simulink model "lee_controller"  (R2021b)
settings: Solver=FixedStepAuto  StartTime=0.0  StopTime=inf  FixedStep=dt  RelTol=1e-3  EnableMultiTasking=on
values from neighbouring files (symbols this model uses):
  dt = 1/250    (= 0.004)    [parameters.m]
  ei = [0,0,0]'    [parameters.m]
  eir = [0,0,0]'    [parameters.m]
  g = 9.81    [parameters.m]
  pitch_offset = 0.028    [parameters.m]
  roll_offset = 0.028    [parameters.m]
  thrust_offset = 0.075    [parameters.m]
  yaw_offset = 0.028    [parameters.m]
undefined symbols (not defined in the file or in its folder): AUX, ddz, dev, DiscIntNeverNeededParam, dz, ep, ev, ew, eyaw, f_ext, fz, Main, pwm_output0, pwm_output1, tau, timestamp, z
libraries: px4lib x47, px4uORBlib x14, px4Sensorslib x1
(part 1 of 2)
settings Model: SimulationMode=external  ExtModeTrigDuration=10  Creator=salvatore  LastModifiedBy=simone
settings SolverCC: PositivePriorityOrder=on
settings DataIOCC: MaxDataPoints=7018
settings OptimizationCC: EnhancedBackFolding=on  PassReuseOutputArgsAs=Individual arguments  ZeroExternalMemoryAtStartup=off  ZeroInternalMemoryAtStartup=off  MaxStackSize=64  OptimizeBlockOrder=speed  DifferentSizesBufferReuse=on  OptimizationCustomize=off  EfficientTunableParamExpr=on
settings DebuggingCC: ParameterTunabilityLossMsg=error
settings HardwareCC: ProdBitPerPointer=32  ProdBitPerSizeT=32  ProdBitPerPtrDiffT=32  ProdLargestAtomicInteger=Long  ProdLargestAtomicFloat=Double  ProdWordSize=32  ProdLongLongMode=on  ProdHWDeviceType=ARM Compatible->ARM Cortex
settings SFSimCC: MATLABDynamicMemAlloc=off  SimTargetLang=C++
settings RTWCC: Description=Embedded Coder  SystemTargetFile=ert.tlc  HardwareBoard=PX4 Pixhawk 4  TLCOptions="-aInlineSetEventsForThisBaseRateFcn=TLC_FALSE -aSuppressMultiTaskScheduler=TLC_FALSE  -aRateBasedStepFcn=0"  TemplateMakefile=ert_default_tmf  Toolchain=GNU Tools for PX4 Autopilots  TargetLang=C++
settings CodeAppCC: ForceParamTrailComments=on  IgnoreCustomStorageClasses=off  OperatorAnnotations=on  SimulinkDataObjDesc=on  SFDataObjDesc=on  InsertBlockDesc=on
settings ERTTargetCC: ExtMode=on  ExtModeTransport=3  ExtModeStaticAlloc=on  ExtModeStaticAllocSize=1024  ExtModeMexFile=ext_xcp  ExtModeMexArgs=1 /dev/ttyUSB0 115200  ExtModeIntrfLevel=Level2 - Open

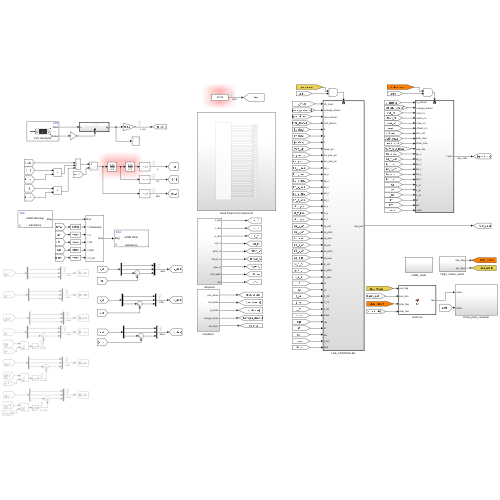
[thumbnail: Simulink's stored preview of the top-level diagram]
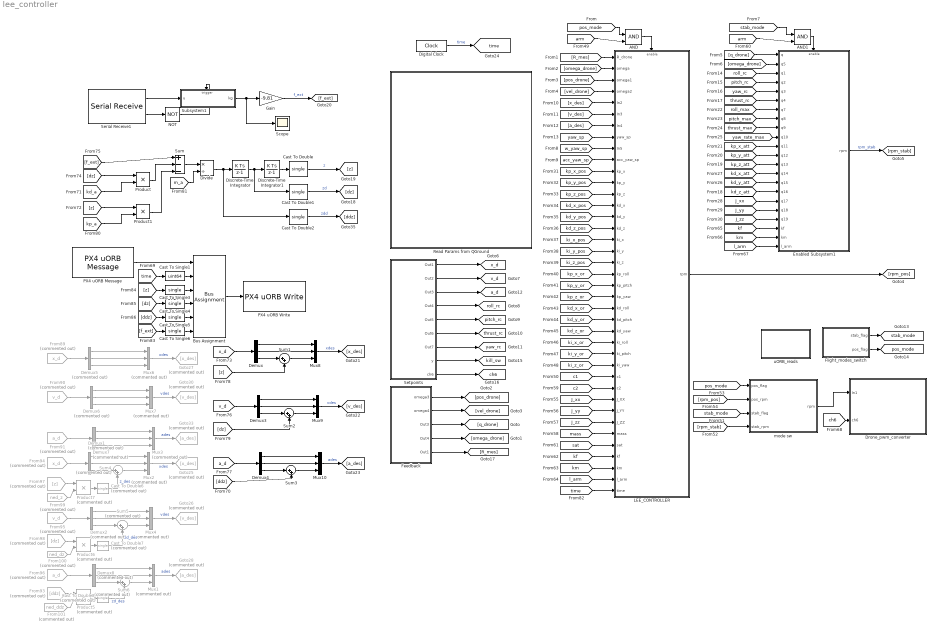
== system lee_controller ==
  AND : Logic  IconShape=distinctive  AllPortsSameDT=off  OutDataTypeStr=boolean
  AND1 : Logic  IconShape=distinctive  AllPortsSameDT=off  OutDataTypeStr=boolean
  Bus Assignment : BusAssignment  AssignedSignals=timestamp,z,dz,ddz,f_ext
  Cast To Double : DataTypeConversion  OutDataTypeStr=single
  Cast To Double1 : DataTypeConversion  OutDataTypeStr=single
  Cast To Double2 : DataTypeConversion  OutDataTypeStr=single
  Cast To Double6 : DataTypeConversion  Commented=on  OutDataTypeStr=single
  Cast To Double7 : DataTypeConversion  Commented=on  OutDataTypeStr=single
  Cast To Double8 : DataTypeConversion  Commented=on  OutDataTypeStr=single
  Cast To Single1 : DataTypeConversion  OutDataTypeStr=uint64
  Cast To Single{3..6} (4 alike) : DataTypeConversion  OutDataTypeStr=single
  Demux : Demux  Outputs=3
  Demux{1..2,5..8} (6 alike) : Demux  Commented=on  Outputs=3
  Demux3 : Demux  Outputs=3
  Demux4 : Demux  Outputs=3
  Digital Clock : DigitalClock  SampleTime=dt
  Discrete-Time Integrator : DiscreteIntegrator  SampleTime=dt  OutDataTypeStr=double  ICPrevOutput=DiscIntNeverNeededParam  ICPrevScaledInput=DiscIntNeverNeededParam
  Discrete-Time Integrator1 : DiscreteIntegrator  SampleTime=dt  OutDataTypeStr=double  ICPrevOutput=DiscIntNeverNeededParam  ICPrevScaledInput=DiscIntNeverNeededParam
  Divide : Product  Inputs=*/  OutDataTypeStr=double
  Drone_pwm_converter : Subsystem
  Enabled Subsystem1 : Subsystem  TreatAsAtomicUnit=on
  Feedback : Subsystem
  Flight_modes_switch : Subsystem
  From100 : From  Commented=on  GotoTag=ned_dz  TagVisibility=global
  From101 : From  Commented=on  GotoTag=ned_ddz  TagVisibility=global
  From89 : From  Commented=on  GotoTag=x_d  TagVisibility=global
  From90 : From  Commented=on  GotoTag=v_d  TagVisibility=global
  From91 : From  Commented=on  GotoTag=a_d  TagVisibility=global
  From93 : From  Commented=on  GotoTag=ddz
  From94 : From  Commented=on  GotoTag=x_d  TagVisibility=global
  From95 : From  Commented=on  GotoTag=v_d  TagVisibility=global
  From96 : From  Commented=on  GotoTag=a_d  TagVisibility=global
  From97 : From  Commented=on  GotoTag=z
  From98 : From  Commented=on  GotoTag=dz
  From99 : From  Commented=on  GotoTag=ned_z  TagVisibility=global
  Gain : Gain  Gain=-9.81
  Goto25 : Goto  Commented=on  GotoTag=x_des
  Goto26 : Goto  Commented=on  GotoTag=v_des
  Goto27 : Goto  Commented=on  GotoTag=x_des
  Goto28 : Goto  Commented=on  GotoTag=a_des
  Goto30 : Goto  Commented=on  GotoTag=v_des
  Goto33 : Goto  Commented=on  GotoTag=a_des
  LEE_CONTROLLER : Subsystem  TreatAsAtomicUnit=on
  Mux{1..4,6..7} (6 alike) : Mux  Commented=on  Inputs=3
  Mux10 : Mux  Inputs=3
  Mux8 : Mux  Inputs=3
  Mux9 : Mux  Inputs=3
  NOT : Logic  Operator=NOT  IconShape=distinctive  AllPortsSameDT=off  OutDataTypeStr=boolean
  PX4 uORB Message : px4uORBlib/PX4 uORB Message  uORBTopic=admittance  SampleTime=dt  selectInstance=admittance
      settings: SourceProductBaseCode=PX4AUTOPILOTS
  PX4 uORB Write : px4uORBlib/PX4 uORB Write  uORBTopic=admittance  selectInstance=admittance  MessageQueueLen=1
      settings: SourceProductBaseCode=PX4AUTOPILOTS
  Product : Product
  Product1 : Product
  Product5 : Product  Commented=on
  Product6 : Product  Commented=on
  Product7 : Product  Commented=on
  Read Params from QGround : Subsystem
  Scope : Scope
  Serial Receive1 : px4lib/Serial Receive  SCIModule=/dev/ttyS2  DataType=int8  DataLength=2  OutputStatus=on  SampleTime=dt  BlockingMode=off  PartialData=off  Timeout=5
      settings: SourceProductBaseCode=PX4AUTOPILOTS
  Setpoints : Subsystem
  Subsystem1 : Subsystem
  Sum : Sum  Inputs=|+--
  Sum1 : Sum  Inputs=|++
  Sum2 : Sum  Inputs=|++
  Sum3 : Sum  Inputs=|++
  Sum4 : Sum  Commented=on  Inputs=|++
  Sum5 : Sum  Commented=on  Inputs=|++
  Sum6 : Sum  Commented=on  Inputs=|++
  mode sw : MATLAB Function  TreatAsAtomicUnit=on
  uORB_reads : Subsystem
  tag scope: a_d=global, ch6=global, kill_sw=global, pitch_rc=global, pos_mode=global, roll_rc=global, stab_mode=global, thrust_rc=global, time=global, v_d=global, x_d=global, yaw_rc=global
  wires:
  [omega_drone] -> LEE_CONTROLLER/2(omega)
  [pos_drone] -> LEE_CONTROLLER/3(omega1)
  [vel_drone] -> LEE_CONTROLLER/4(omega2)
  [omega_drone] -> Enabled Subsystem1/2(q5)
  Enabled Subsystem1/1(rpm) -> [rpm_stab]  "rpm_stab"
  [x_des] -> LEE_CONTROLLER/5(In2)
  [v_des] -> LEE_CONTROLLER/6(In3)
  [a_des] -> LEE_CONTROLLER/7(In4)
  Setpoints/2(Out2) -> [v_d]
  Setpoints/1(Out1) -> [x_d]
  Setpoints/3(Out3) -> [a_d]
  Setpoints/4(Out4) -> [roll_rc]
  Setpoints/5(Out5) -> [pitch_rc]
  Setpoints/7(Out7) -> [yaw_rc]
  Setpoints/6(Out6) -> [thrust_rc]
  [roll_rc] -> Enabled Subsystem1/3(q1)
  [pitch_rc] -> Enabled Subsystem1/4(q2)
  [yaw_rc] -> Enabled Subsystem1/5(q3)
  [thrust_rc] -> Enabled Subsystem1/6(q4)
  Flight_modes_switch/1(stab_flag) -> [stab_mode]
  Flight_modes_switch/2(pos_flag) -> [pos_mode]
  [q_drone] -> Enabled Subsystem1/1(q)
  Setpoints/8(y) -> [kill_sw]
  [roll_max] -> Enabled Subsystem1/7(q7)
  [pitch_max] -> Enabled Subsystem1/8(q8)
  [thrust_max] -> Enabled Subsystem1/9(q9)
  [yaw_rate_max] -> Enabled Subsystem1/10(q10)
  [kp_x_att] -> Enabled Subsystem1/11(q11)
  [kp_y_att] -> Enabled Subsystem1/12(q12)
  [kp_z_att] -> Enabled Subsystem1/13(q13)
  [kd_x_att] -> Enabled Subsystem1/14(q14)
  [kd_y_att] -> Enabled Subsystem1/15(q15)
  [kd_z_att] -> Enabled Subsystem1/16(q16)
  [J_zz] -> Enabled Subsystem1/19(q19)
  [J_yy] -> Enabled Subsystem1/18(q18)
  [J_xx] -> Enabled Subsystem1/17(q17)
  [kp_x_pos] -> LEE_CONTROLLER/11(kp_x)
  [kp_y_pos] -> LEE_CONTROLLER/12(kp_y)
  [kp_z_pos] -> LEE_CONTROLLER/13(kp_z)
  [kd_x_pos] -> LEE_CONTROLLER/14(kd_x)
  [kd_y_pos] -> LEE_CONTROLLER/15(kd_y)
  [kd_z_pos] -> LEE_CONTROLLER/16(kd_z)
  [ki_x_pos] -> LEE_CONTROLLER/17(ki_x)
  [ki_y_pos] -> LEE_CONTROLLER/18(ki_y)
  [ki_z_pos] -> LEE_CONTROLLER/19(ki_z)
  [kp_x_or] -> LEE_CONTROLLER/20("kp_roll\t")
  [kp_y_or] -> LEE_CONTROLLER/21(kp_pitch)
  [kp_z_or] -> LEE_CONTROLLER/22(kp_yaw)
  [kd_x_or] -> LEE_CONTROLLER/23(kd_roll)
  [kd_y_or] -> LEE_CONTROLLER/24(kd_pitch)
  [kd_z_or] -> LEE_CONTROLLER/25(kd_yaw)
  [ki_x_or] -> LEE_CONTROLLER/26(ki_roll)
  [ki_y_or] -> LEE_CONTROLLER/27(ki_pitch)
  [ki_z_or] -> LEE_CONTROLLER/28(ki_yaw)
  [c1] -> LEE_CONTROLLER/29(c1)
  [stab_mode] -> mode sw/3(stab_flag)
  [rpm_stab] -> mode sw/4(stab_rpm)
  [rpm_pos] -> mode sw/2(pos_rpm)
  [pos_mode] -> mode sw/1(pos_flag)
  mode sw/1(rpm) -> Drone_pwm_converter/1(In1)
  [J_yy] -> LEE_CONTROLLER/32(J_YY)
  [J_xx] -> LEE_CONTROLLER/31(J_XX)
  [J_zz] -> LEE_CONTROLLER/33(J_ZZ)
  [c2] -> LEE_CONTROLLER/30(c2)
  [mass] -> LEE_CONTROLLER/34("mass ")
  Feedback/1(omega3) -> [pos_drone]
  Feedback/3(Out3) -> [q_drone]
  Feedback/4(Out4) -> [omega_drone]
  Feedback/2(omega4) -> [vel_drone]
  [yaw_sp] -> LEE_CONTROLLER/8(yaw_sp)
  [w_yaw_sp] -> LEE_CONTROLLER/9(In5)
  [acc_yaw_sp] -> LEE_CONTROLLER/10(acc_yaw_sp)
  Feedback/5(Out1) -> [R_mes]
  [R_mes] -> LEE_CONTROLLER/1(R_drone)
  LEE_CONTROLLER/1(rpm) -> [rpm_pos]
  AND/1 -> LEE_CONTROLLER/Enable
  [pos_mode] -> AND/1
  [arm] -> AND/2
  AND1/1 -> Enabled Subsystem1/Enable
  [arm] -> AND1/2
  [stab_mode] -> AND1/1
  [sat] -> LEE_CONTROLLER/35(sat)
  [kf] -> LEE_CONTROLLER/36(kf)
  [km] -> LEE_CONTROLLER/37(km)
  [l_arm] -> LEE_CONTROLLER/38(l_arm)
  [kf] -> Enabled Subsystem1/20(kf)
  [km] -> Enabled Subsystem1/21(km)
  [l_arm] -> Enabled Subsystem1/22(l_arm)
  Setpoints/9(ch6) -> [ch6]
  [ch6] -> Drone_pwm_converter/2(ch6)
  Sum1/1 -> Mux8/3
  Demux3/3 -> Sum2/1
  Demux4/1 -> Mux10/1
  [m_a] -> Divide/2
  [f_ext] -> Sum/1
  Demux/1 -> Mux8/1
  Gain/1 -> [f_ext]  "f_ext"
  Sum3/1 -> Mux10/3
  Divide/1 -> Cast To Double2/1, Discrete-Time Integrator/1
  [dz] -> Product/1
  NOT/1 -> Subsystem1/Trigger
  Serial Receive1/2 -> NOT/1
  Sum2/1 -> Mux9/3
  [x_d] -> Demux/1
  Mux10/1 -> [a_des]  "ades"
  Discrete-Time Integrator/1 -> Discrete-Time Integrator1/1, Cast To Double1/1
  Demux/2 -> Mux8/2
  Cast To Single3/1 -> Bus Assignment/3
  [dz] -> Cast To Single4/1
  Sum/1 -> Divide/1
  Cast To Single4/1 -> Bus Assignment/4
  Demux3/1 -> Mux9/1
  [z] -> Cast To Single3/1
  Cast To Single5/1 -> Bus Assignment/5
  [a_d] -> Demux4/1
  Demux4/3 -> Sum3/1
  Subsystem1/1(kg) -> Scope/1, Gain/1
  Bus Assignment/1 -> PX4 uORB Write/1
  Demux4/2 -> Mux10/2
  [ddz] -> Cast To Single5/1
  Cast To Single6/1 -> Bus Assignment/6
  Demux3/2 -> Mux9/2
  [f_ext] -> Cast To Single6/1
  [kd_a] -> Product/2
  Product/1 -> Sum/2
  Mux8/1 -> [x_des]  "xdes"
  Product1/1 -> Sum/3
  PX4 uORB Message/1 -> Bus Assignment/1
  [z] -> Product1/1
  Mux9/1 -> [v_des]  "vdes"
  [kp_a] -> Product1/2
  Serial Receive1/1 -> Subsystem1/1(u)
  [v_d] -> Demux3/1
  Demux/3 -> Sum1/1
  Demux7/2 -> Mux3/2
  Mux6/1 -> Goto27/1  "xdes"
  From90/1 -> Demux6/1
  Demux5/1 -> Mux6/1
  Demux6/3 -> Mux7/3
  Demux5/2 -> Mux6/2
  From91/1 -> Demux7/1
  Demux7/3 -> Mux3/3
  Mux3/1 -> Goto33/1  "ades"
  Demux6/1 -> Mux7/1
  From89/1 -> Demux5/1
  Demux6/2 -> Mux7/2
  Demux5/3 -> Mux6/3
  Demux7/1 -> Mux3/1
  Mux7/1 -> Goto30/1  "vdes"
  Discrete-Time Integrator1/1 -> Cast To Double/1
  Cast To Double/1 -> [z]  "z"
  Cast To Double1/1 -> [dz]  "zd"
  Cast To Double2/1 -> [ddz]  "zdd"
  Digital Clock/1 -> [time]  "time"
  [time] -> Cast To Single1/1
  Cast To Single1/1 -> Bus Assignment/2
  [time] -> LEE_CONTROLLER/39(time)
  [z] -> Sum1/2
  [dz] -> Sum2/2
  [ddz] -> Sum3/2
  Product5/1 -> Cast To Double8/1
  Product7/1 -> Cast To Double6/1
  Demux8/1 -> Mux1/1
  From93/1 -> Product5/1
  Sum6/1 -> Mux1/3
  From94/1 -> Demux1/1
  Mux4/1 -> Goto26/1  "vdes"
  Cast To Double6/1 -> Sum4/2  "z_des"
  Demux2/2 -> Mux4/2
  Demux8/2 -> Mux1/2
  Product6/1 -> Cast To Double7/1
  Demux1/3 -> Sum4/1
  From97/1 -> Product7/1
  Demux1/2 -> Mux2/2
  From95/1 -> Demux2/1
  From99/1 -> Product7/2
  Sum4/1 -> Mux2/3
  Demux2/1 -> Mux4/1
  From100/1 -> Product6/2
  Sum5/1 -> Mux4/3
  Mux1/1 -> Goto28/1  "ades"
  From98/1 -> Product6/1
  From101/1 -> Product5/2
  Demux2/3 -> Sum5/1
  Cast To Double7/1 -> Sum5/2  "zd_des"
  From96/1 -> Demux8/1
  Cast To Double8/1 -> Sum6/2  "zd_des"
  Demux1/1 -> Mux2/1
  Demux8/3 -> Sum6/1
  Mux2/1 -> Goto25/1  "xdes"

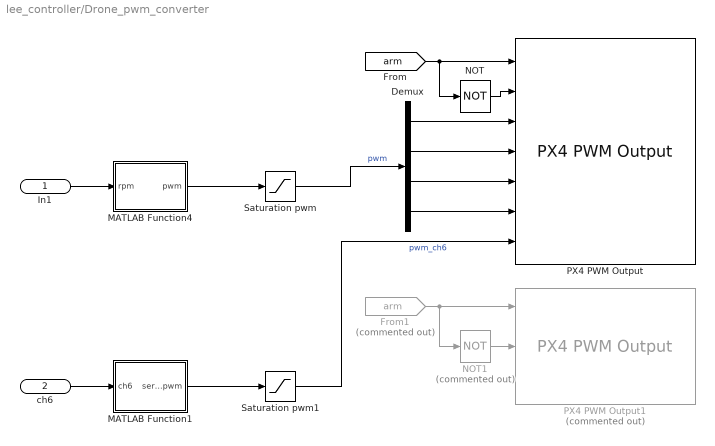
== system lee_controller/Drone_pwm_converter ==
  In1 : Inport
  ch6 : Inport  Port=2
  Demux : Demux
  From1 : From  Commented=on  GotoTag=arm  TagVisibility=global
  MATLAB Function1 : MATLAB Function  TreatAsAtomicUnit=on
  MATLAB Function4 : MATLAB Function  TreatAsAtomicUnit=on
  NOT : Logic  Operator=NOT  IconShape=distinctive  AllPortsSameDT=off  OutDataTypeStr=boolean
  NOT1 : Logic  Commented=on  Operator=NOT  IconShape=distinctive  AllPortsSameDT=off  OutDataTypeStr=boolean
  PX4 PWM Output : px4lib/PX4 PWM Output  pwmDevice=Main (/dev/pwm_output0)  pwmChannel1_=on  pwmChannel2_=on  pwmChannel3_=on  pwmChannel4_=on  pwmChannel5_=off  pwmChannel6_=off  pwmChannel7_=off  pwmChannel8_=on  forceTerminateFailsafe=off  outputErrorStatus=off
      settings: SourceProductBaseCode=PX4AUTOPILOTS
  PX4 PWM Output1 : px4lib/PX4 PWM Output  Commented=on  pwmDevice=AUX (/dev/pwm_output1)  pwmChannel1_=off  pwmChannel2_=off  pwmChannel3_=on  pwmChannel4_=off  pwmChannel5_=off  pwmChannel6_=off  pwmChannel7_=off  pwmChannel8_=off  forceTerminateFailsafe=off  outputErrorStatus=off
      settings: SourceProductBaseCode=PX4AUTOPILOTS
  Saturation pwm : Saturate  UpperLimit=2000  LowerLimit=1000  LinearizeAsGain=off
  Saturation pwm1 : Saturate  UpperLimit=2000  LowerLimit=1000  LinearizeAsGain=off
  wires:
  NOT/1 -> PX4 PWM Output/2
  [arm] -> PX4 PWM Output/1, NOT/1
  Demux/4 -> PX4 PWM Output/6
  In1/1 -> MATLAB Function4/1(rpm)
  MATLAB Function4/1(pwm) -> Saturation pwm/1
  Demux/2 -> PX4 PWM Output/4
  Demux/3 -> PX4 PWM Output/5
  Demux/1 -> PX4 PWM Output/3
  Saturation pwm/1 -> Demux/1  "pwm"
  From1/1 -> NOT1/1, PX4 PWM Output1/1
  NOT1/1 -> PX4 PWM Output1/2
  ch6/1 -> MATLAB Function1/1(ch6)
  Saturation pwm1/1 -> PX4 PWM Output/7  "pwm_ch6"
  MATLAB Function1/1(servo_pwm) -> Saturation pwm1/1

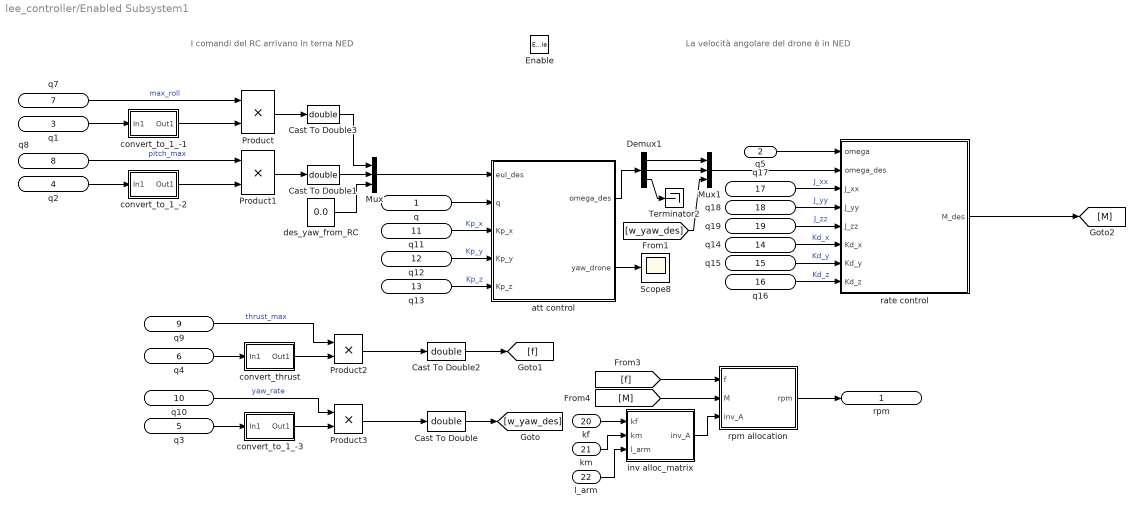
== system lee_controller/Enabled Subsystem1 ==
  note: La velocità angolare del drone è in NED
  note: I comandi del RC arrivano in terna NED
  q : Inport
  q5 : Inport  Port=2
  q1 : Inport  Port=3
  q2 : Inport  Port=4
  q3 : Inport  Port=5
  q4 : Inport  Port=6
  q7 : Inport  Port=7
  q8 : Inport  Port=8
  q9 : Inport  Port=9
  q10 : Inport  Port=10
  q11 : Inport  Port=11
  q12 : Inport  Port=12
  q13 : Inport  Port=13
  q14 : Inport  Port=14
  q15 : Inport  Port=15
  q16 : Inport  Port=16
  q17 : Inport  Port=17
  q18 : Inport  Port=18
  q19 : Inport  Port=19
  kf : Inport  Port=20
  km : Inport  Port=21
  l_arm : Inport  Port=22
  Enable : EnablePort
  Cast To Double{,1..3} (4 alike) : DataTypeConversion  OutDataTypeStr=double
  Demux1 : Demux  Outputs=3
  Mux : Mux  Inputs=3
  Mux1 : Mux  Inputs=3
  Product{,1..3} (4 alike) : Product
  Scope8 : Scope
  Terminator2 : Terminator
  att control : MATLAB Function  TreatAsAtomicUnit=on
  convert_thrust : Subsystem
  convert_to_1_-1 : Subsystem
  convert_to_1_-2 : Subsystem
  convert_to_1_-3 : Subsystem
  des_yaw_from_RC : Constant  Value=0.0  SampleTime=-1
  inv alloc_matrix : MATLAB Function  TreatAsAtomicUnit=on
  rate control : MATLAB Function  TreatAsAtomicUnit=on
  rpm allocation : MATLAB Function  TreatAsAtomicUnit=on
  rpm : Outport
  wires:
  rpm allocation/1(rpm) -> rpm/1
  q4/1 -> convert_thrust/1(In1)
  convert_to_1_-3/1(Out1) -> Product3/2
  q2/1 -> convert_to_1_-2/1(In1)
  [f] -> rpm allocation/1(f)
  convert_thrust/1(Out1) -> Product2/2
  convert_to_1_-2/1(Out1) -> Product1/2
  q1/1 -> convert_to_1_-1/1(In1)
  convert_to_1_-1/1(Out1) -> Product/2
  q3/1 -> convert_to_1_-3/1(In1)
  [M] -> rpm allocation/2(M)
  q5/1 -> rate control/1(omega)
  rate control/1(M_des) -> [M]
  Product2/1 -> Cast To Double2/1
  Product/1 -> Cast To Double3/1
  att control/1(omega_des) -> Demux1/1
  Demux1/1 -> Mux1/1
  Demux1/2 -> Mux1/2
  Demux1/3 -> Terminator2/1
  [w_yaw_des] -> Mux1/3
  Mux1/1 -> rate control/2(omega_des)
  Cast To Double1/1 -> Mux/2
  Product3/1 -> Cast To Double/1
  Cast To Double/1 -> [w_yaw_des]
  Mux/1 -> att control/1(eul_des)
  Cast To Double2/1 -> [f]
  Cast To Double3/1 -> Mux/1
  q7/1 -> Product/1  "max_roll"
  Product1/1 -> Cast To Double1/1
  q10/1 -> Product3/1  "yaw_rate"
  q/1 -> att control/2(q)
  q8/1 -> Product1/1  "pitch_max"
  q9/1 -> Product2/1  "thrust_max"
  q11/1 -> att control/3(Kp_x)  "Kp_x"
  q12/1 -> att control/4(Kp_y)  "Kp_y"
  q13/1 -> att control/5(Kp_z)  "Kp_z"
  q14/1 -> rate control/6(Kd_x)  "Kd_x"
  q15/1 -> rate control/7(Kd_y)  "Kd_y"
  q16/1 -> rate control/8(Kd_z)  "Kd_z"
  q17/1 -> rate control/3(J_xx)  "J_xx"
  q18/1 -> rate control/4(J_yy)  "J_yy"
  q19/1 -> rate control/5(J_zz)  "J_zz"
  des_yaw_from_RC/1 -> Mux/3
  att control/2(yaw_drone) -> Scope8/1
  kf/1 -> inv alloc_matrix/1(kf)
  km/1 -> inv alloc_matrix/2(km)
  l_arm/1 -> inv alloc_matrix/3(l_arm)
  inv alloc_matrix/1(inv_A) -> rpm allocation/3(inv_A)

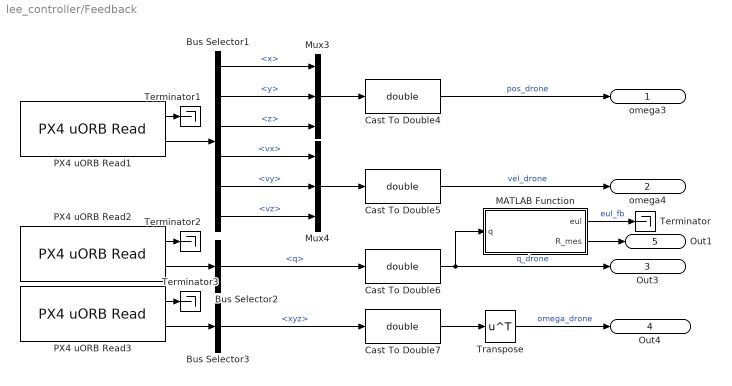
== system lee_controller/Feedback ==
  Bus Selector1 : BusSelector  OutputSignals=x,y,z,vx,vy,vz
  Bus Selector2 : BusSelector  OutputSignals=q
  Bus Selector3 : BusSelector  OutputSignals=xyz
  Cast To Double{4..7} (4 alike) : DataTypeConversion  OutDataTypeStr=double
  MATLAB Function : MATLAB Function  TreatAsAtomicUnit=on
  Mux3 : Mux  Inputs=3
  Mux4 : Mux  Inputs=3
  PX4 uORB Read1 : px4uORBlib/PX4 uORB Read  uORBTopic=vehicle_local_position  selectInstance=vehicle_local_position  SampleTime=dt  BlockingMode=off  BlockTimeout=1e-3
      settings: SourceProductBaseCode=PX4AUTOPILOTS
  PX4 uORB Read2 : px4uORBlib/PX4 uORB Read  uORBTopic=vehicle_attitude  selectInstance=vehicle_attitude  SampleTime=dt  BlockingMode=off  BlockTimeout=1e-3
      settings: SourceProductBaseCode=PX4AUTOPILOTS
  PX4 uORB Read3 : px4uORBlib/PX4 uORB Read  uORBTopic=vehicle_angular_velocity  selectInstance=vehicle_angular_velocity  SampleTime=dt  BlockingMode=off  BlockTimeout=1e-3
      settings: SourceProductBaseCode=PX4AUTOPILOTS
  Terminator{,1..3} (4 alike) : Terminator
  Transpose : Math  Operator=transpose  SaturateOnIntegerOverflow=on
  omega3 : Outport
  omega4 : Outport  Port=2
  Out3 : Outport  Port=3
  Out4 : Outport  Port=4
  Out1 : Outport  Port=5
  wires:
  PX4 uORB Read1/2 -> Bus Selector1/1
  PX4 uORB Read2/2 -> Bus Selector2/1
  PX4 uORB Read3/2 -> Bus Selector3/1
  PX4 uORB Read1/1 -> Terminator1/1
  PX4 uORB Read2/1 -> Terminator2/1
  PX4 uORB Read3/1 -> Terminator3/1
  Cast To Double4/1 -> omega3/1  "pos_drone"
  Mux3/1 -> Cast To Double4/1
  Bus Selector1/3 -> Mux3/3  "<z>"
  Bus Selector1/1 -> Mux3/1  "<x>"
  Bus Selector1/2 -> Mux3/2  "<y>"
  Cast To Double5/1 -> omega4/1  "vel_drone"
  Mux4/1 -> Cast To Double5/1
  Bus Selector1/6 -> Mux4/3  "<vz>"
  Bus Selector1/4 -> Mux4/1  "<vx>"
  Bus Selector1/5 -> Mux4/2  "<vy>"
  Bus Selector2/1 -> Cast To Double6/1  "<q>"
  Cast To Double6/1 -> Out3/1, MATLAB Function/1(q)  "q_drone"
  Bus Selector3/1 -> Cast To Double7/1  "<xyz>"
  Cast To Double7/1 -> Transpose/1
  Transpose/1 -> Out4/1  "omega_drone"
  MATLAB Function/1(eul) -> Terminator/1  "eul_fb"
  MATLAB Function/2(R_mes) -> Out1/1

== system lee_controller/Flight_modes_switch ==
  MATLAB Function : MATLAB Function  TreatAsAtomicUnit=on
  stab_flag : Outport
  pos_flag : Outport  Port=2
  wires:
  MATLAB Function/1(stab_flag) -> stab_flag/1  "stab_flag"
  [flight_mode] -> MATLAB Function/1(flight_mode)
  MATLAB Function/2(pos_flag) -> pos_flag/1  "pos_flag"

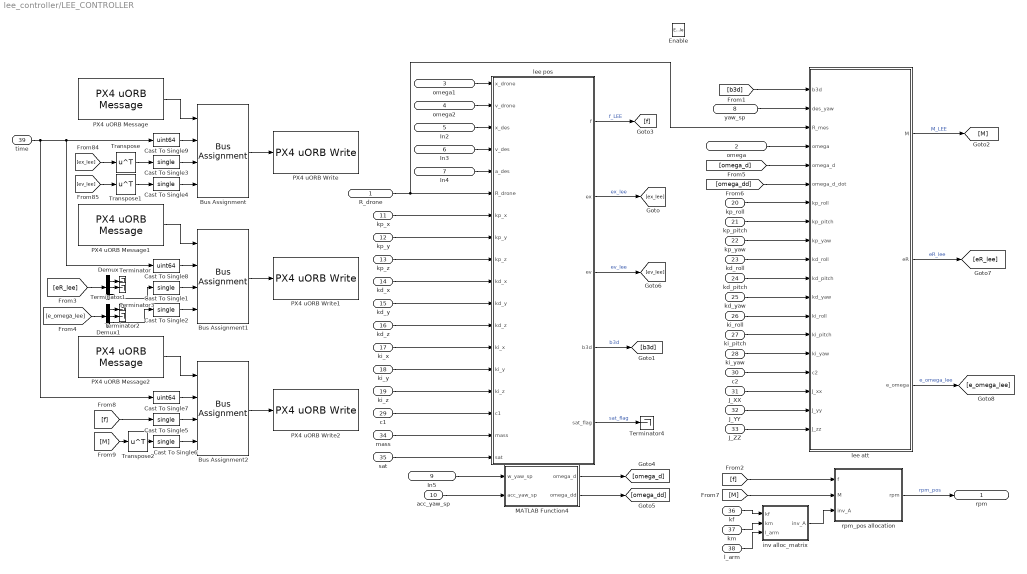
== system lee_controller/LEE_CONTROLLER ==
  R_drone : Inport
  omega : Inport  Port=2
  omega1 : Inport  Port=3
  omega2 : Inport  Port=4
  In2 : Inport  Port=5
  In3 : Inport  Port=6
  In4 : Inport  Port=7
  yaw_sp : Inport  Port=8
  In5 : Inport  Port=9
  acc_yaw_sp : Inport  Port=10
  kp_x : Inport  Port=11
  kp_y : Inport  Port=12
  kp_z : Inport  Port=13
  kd_x : Inport  Port=14
  kd_y : Inport  Port=15
  kd_z : Inport  Port=16
  ki_x : Inport  Port=17
  ki_y : Inport  Port=18
  ki_z : Inport  Port=19
  "kp_roll\t" : Inport  Port=20
  kp_pitch : Inport  Port=21
  kp_yaw : Inport  Port=22
  kd_roll : Inport  Port=23
  kd_pitch : Inport  Port=24
  kd_yaw : Inport  Port=25
  ki_roll : Inport  Port=26
  ki_pitch : Inport  Port=27
  ki_yaw : Inport  Port=28
  c1 : Inport  Port=29
  c2 : Inport  Port=30
  J_XX : Inport  Port=31
  J_YY : Inport  Port=32
  J_ZZ : Inport  Port=33
  "mass " : Inport  Port=34
  sat : Inport  Port=35
  kf : Inport  Port=36
  km : Inport  Port=37
  l_arm : Inport  Port=38
  time : Inport  Port=39
  Enable : EnablePort
  Bus Assignment : BusAssignment  AssignedSignals=timestamp,ep,ev
  Bus Assignment1 : BusAssignment  AssignedSignals=timestamp,eyaw,ew
  Bus Assignment2 : BusAssignment  AssignedSignals=timestamp,fz,tau
  Cast To Single{1..6} (6 alike) : DataTypeConversion  OutDataTypeStr=single
  Cast To Single7 : DataTypeConversion  OutDataTypeStr=uint64
  Cast To Single8 : DataTypeConversion  OutDataTypeStr=uint64
  Cast To Single9 : DataTypeConversion  OutDataTypeStr=uint64
  Demux : Demux  Outputs=3
  Demux1 : Demux  Outputs=3
  MATLAB Function4 : MATLAB Function  TreatAsAtomicUnit=on
  PX4 uORB Message : px4uORBlib/PX4 uORB Message  uORBTopic=linear_err  SampleTime=dt  selectInstance=linear_err
      settings: SourceProductBaseCode=PX4AUTOPILOTS
  PX4 uORB Message1 : px4uORBlib/PX4 uORB Message  uORBTopic=ang_err  SampleTime=dt  selectInstance=ang_err
      settings: SourceProductBaseCode=PX4AUTOPILOTS
  PX4 uORB Message2 : px4uORBlib/PX4 uORB Message  uORBTopic=act_wrench  SampleTime=dt  selectInstance=act_wrench
      settings: SourceProductBaseCode=PX4AUTOPILOTS
  PX4 uORB Write : px4uORBlib/PX4 uORB Write  uORBTopic=linear_err  selectInstance=linear_err  MessageQueueLen=1
      settings: SourceProductBaseCode=PX4AUTOPILOTS
  PX4 uORB Write1 : px4uORBlib/PX4 uORB Write  uORBTopic=ang_err  selectInstance=ang_err  MessageQueueLen=1
      settings: SourceProductBaseCode=PX4AUTOPILOTS
  PX4 uORB Write2 : px4uORBlib/PX4 uORB Write  uORBTopic=act_wrench  selectInstance=act_wrench  MessageQueueLen=1
      settings: SourceProductBaseCode=PX4AUTOPILOTS
  Terminator{,1..4} (5 alike) : Terminator
  Transpose : Math  Operator=transpose  SaturateOnIntegerOverflow=on
  Transpose1 : Math  Operator=transpose  SaturateOnIntegerOverflow=on
  Transpose2 : Math  Operator=transpose  SaturateOnIntegerOverflow=on
  inv alloc_matrix : MATLAB Function  TreatAsAtomicUnit=on
  lee att : MATLAB Function  TreatAsAtomicUnit=on
  lee pos : MATLAB Function  TreatAsAtomicUnit=on
  rpm_pos allocation : MATLAB Function  TreatAsAtomicUnit=on
  rpm : Outport
  wires:
  lee pos/4(b3d) -> [b3d]  "b3d"
  omega/1 -> lee att/4(omega)
  [omega_dd] -> lee att/6(omega_d_dot)
  omega2/1 -> lee pos/2(v_drone)
  omega1/1 -> lee pos/1(x_drone)
  In2/1 -> lee pos/3(x_des)
  [omega_d] -> lee att/5(omega_d)
  lee att/2(eR) -> [eR_lee]  "eR_lee"
  [b3d] -> lee att/1(b3d)
  lee pos/1(f) -> [f]  "f_LEE"
  In4/1 -> lee pos/5(a_des)
  lee att/1(M) -> [M]  "M_LEE"
  In3/1 -> lee pos/4(v_des)
  kp_x/1 -> lee pos/7(kp_x)
  kp_y/1 -> lee pos/8(kp_y)
  kp_z/1 -> lee pos/9(kp_z)
  kd_x/1 -> lee pos/10(kd_x)
  kd_y/1 -> lee pos/11(kd_y)
  ki_x/1 -> lee pos/13(ki_x)
  ki_y/1 -> lee pos/14(ki_y)
  ki_z/1 -> lee pos/15(ki_z)
  c1/1 -> lee pos/16(c1)
  kd_z/1 -> lee pos/12(kd_z)
  "kp_roll\t"/1 -> lee att/7(kp_roll)
  kp_pitch/1 -> lee att/8(kp_pitch)
  kp_yaw/1 -> lee att/9(kp_yaw)
  kd_roll/1 -> lee att/10(kd_roll)
  kd_pitch/1 -> lee att/11(kd_pitch)
  kd_yaw/1 -> lee att/12(kd_yaw)
  ki_roll/1 -> lee att/13(ki_roll)
  ki_pitch/1 -> lee att/14(ki_pitch)
  ki_yaw/1 -> lee att/15(ki_yaw)
  c2/1 -> lee att/16(c2)
  J_XX/1 -> lee att/17(J_xx)
  J_YY/1 -> lee att/18(J_yy)
  J_ZZ/1 -> lee att/19(J_zz)
  "mass "/1 -> lee pos/17(mass)
  MATLAB Function4/1(omega_d) -> [omega_d]
  lee pos/2(ex) -> [ex_lee]  "ex_lee"
  lee pos/3(ev) -> [ev_lee]  "ev_lee"
  lee att/3(e_omega) -> [e_omega_lee]  "e_omega_lee"
  In5/1 -> MATLAB Function4/1(w_yaw_sp)
  yaw_sp/1 -> lee att/2(des_yaw)
  acc_yaw_sp/1 -> MATLAB Function4/2(acc_yaw_sp)
  MATLAB Function4/2(omega_dd) -> [omega_dd]
  R_drone/1 -> lee att/3(R_mes), lee pos/6(R_drone)
  [M] -> rpm_pos allocation/2(M)
  rpm_pos allocation/1(rpm) -> rpm/1  "rpm_pos"
  [f] -> rpm_pos allocation/1(f)
  sat/1 -> lee pos/18(sat)
  lee pos/5(sat_flag) -> Terminator4/1  "sat_flag"
  inv alloc_matrix/1(inv_A) -> rpm_pos allocation/3(inv_A)
  kf/1 -> inv alloc_matrix/1(kf)
  km/1 -> inv alloc_matrix/2(km)
  l_arm/1 -> inv alloc_matrix/3(l_arm)
  PX4 uORB Message/1 -> Bus Assignment/1
  Bus Assignment/1 -> PX4 uORB Write/1
  Cast To Single3/1 -> Bus Assignment/3
  Cast To Single4/1 -> Bus Assignment/4
  Cast To Single2/1 -> Bus Assignment1/4
  Cast To Single1/1 -> Bus Assignment1/3
  Bus Assignment1/1 -> PX4 uORB Write1/1
  PX4 uORB Message1/1 -> Bus Assignment1/1
  [f] -> Cast To Single5/1
  PX4 uORB Message2/1 -> Bus Assignment2/1
  Bus Assignment2/1 -> PX4 uORB Write2/1
  Cast To Single5/1 -> Bus Assignment2/3
  Cast To Single6/1 -> Bus Assignment2/4
  [eR_lee] -> Demux/1
  [e_omega_lee] -> Demux1/1
  Demux1/3 -> Cast To Single2/1
  Demux/3 -> Cast To Single1/1
  Demux/1 -> Terminator/1
  Demux/2 -> Terminator1/1
  Demux1/1 -> Terminator2/1
  Demux1/2 -> Terminator3/1
  Transpose/1 -> Cast To Single3/1
  Transpose1/1 -> Cast To Single4/1
  [ev_lee] -> Transpose1/1
  [ex_lee] -> Transpose/1
  [M] -> Transpose2/1
  Transpose2/1 -> Cast To Single6/1
  time/1 -> Cast To Single8/1, Cast To Single9/1, Cast To Single7/1
  Cast To Single7/1 -> Bus Assignment2/2
  Cast To Single8/1 -> Bus Assignment1/2
  Cast To Single9/1 -> Bus Assignment/2

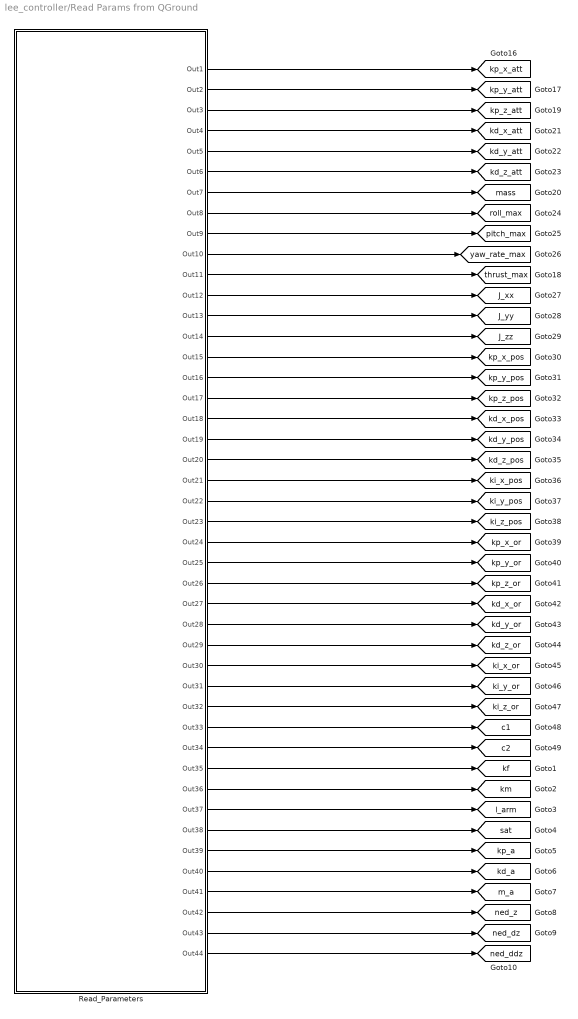
== system lee_controller/Read Params from QGround ==
  Read_Parameters : Subsystem
  tag scope: J_xx=global, J_yy=global, J_zz=global, c1=global, c2=global, kd_a=global, kd_x_att=global, kd_x_or=global, kd_x_pos=global, kd_y_att=global, kd_y_or=global, kd_y_pos=global, kd_z_att=global, kd_z_or=global, kd_z_pos=global, kf=global, ki_x_or=global, ki_x_pos=global, ki_y_or=global, ki_y_pos=global, ki_z_or=global, ki_z_pos=global, km=global, kp_a=global, kp_x_att=global, kp_x_or=global, kp_x_pos=global, kp_y_att=global, kp_y_or=global, kp_y_pos=global, kp_z_att=global, kp_z_or=global, kp_z_pos=global, l_arm=global, m_a=global, mass=global, ned_ddz=global, ned_dz=global, ned_z=global, pitch_max=global, roll_max=global, sat=global, thrust_max=global, yaw_rate_max=global
  wires:
  Read_Parameters/26(Out26) -> [kp_z_or]
  Read_Parameters/19(Out19) -> [kd_y_pos]
  Read_Parameters/15(Out15) -> [kp_x_pos]
  Read_Parameters/32(Out32) -> [ki_z_or]
  Read_Parameters/18(Out18) -> [kd_x_pos]
  Read_Parameters/12(Out12) -> [J_xx]
  Read_Parameters/28(Out28) -> [kd_y_or]
  Read_Parameters/4(Out4) -> [kd_x_att]
  Read_Parameters/23(Out23) -> [ki_z_pos]
  Read_Parameters/27(Out27) -> [kd_x_or]
  Read_Parameters/29(Out29) -> [kd_z_or]
  Read_Parameters/20(Out20) -> [kd_z_pos]
  Read_Parameters/21(Out21) -> [ki_x_pos]
  Read_Parameters/13(Out13) -> [J_yy]
  Read_Parameters/5(Out5) -> [kd_y_att]
  Read_Parameters/6(Out6) -> [kd_z_att]
  Read_Parameters/34(Out34) -> [c2]
  Read_Parameters/17(Out17) -> [kp_z_pos]
  Read_Parameters/14(Out14) -> [J_zz]
  Read_Parameters/10(Out10) -> [yaw_rate_max]
  Read_Parameters/25(Out25) -> [kp_y_or]
  Read_Parameters/8(Out8) -> [roll_max]
  Read_Parameters/16(Out16) -> [kp_y_pos]
  Read_Parameters/31(Out31) -> [ki_y_or]
  Read_Parameters/30(Out30) -> [ki_x_or]
  Read_Parameters/11(Out11) -> [thrust_max]
  Read_Parameters/33(Out33) -> [c1]
  Read_Parameters/22(Out22) -> [ki_y_pos]
  Read_Parameters/24(Out24) -> [kp_x_or]
  Read_Parameters/7(Out7) -> [mass]
  Read_Parameters/2(Out2) -> [kp_y_att]
  Read_Parameters/3(Out3) -> [kp_z_att]
  Read_Parameters/1(Out1) -> [kp_x_att]
  Read_Parameters/9(Out9) -> [pitch_max]
  Read_Parameters/35(Out35) -> [kf]
  Read_Parameters/36(Out36) -> [km]
  Read_Parameters/37(Out37) -> [l_arm]
  Read_Parameters/38(Out38) -> [sat]
  Read_Parameters/39(Out39) -> [kp_a]
  Read_Parameters/40(Out40) -> [kd_a]
  Read_Parameters/41(Out41) -> [m_a]
  Read_Parameters/42(Out42) -> [ned_z]
  Read_Parameters/43(Out43) -> [ned_dz]
  Read_Parameters/44(Out44) -> [ned_ddz]

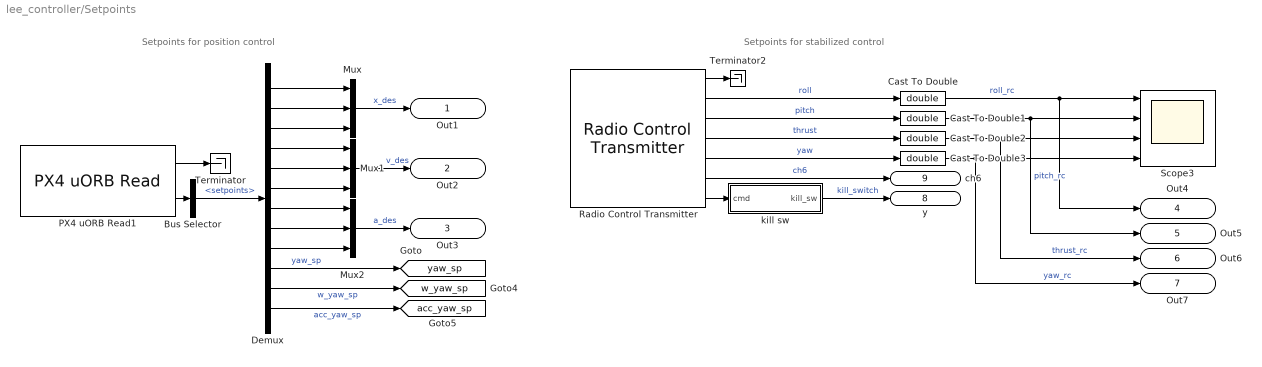
== system lee_controller/Setpoints ==
  note: Setpoints for stabilized control
  note: Setpoints for position control
  Bus Selector : BusSelector  OutputSignals=setpoints
  Cast To Double{,1..3} (4 alike) : DataTypeConversion  OutDataTypeStr=double
  Demux : Demux  Outputs=12
  Mux : Mux  Inputs=3
  Mux1 : Mux  Inputs=3
  Mux2 : Mux  Inputs=3
  PX4 uORB Read1 : px4uORBlib/PX4 uORB Read  uORBTopic=traj_setpoint  selectInstance=traj_setpoint  SampleTime=dt  BlockingMode=off  BlockTimeout=1e-3
      settings: SourceProductBaseCode=PX4AUTOPILOTS
  Radio Control Transmitter : px4Sensorslib/Radio Control Transmitter  channel1=on  channel2=on  channel3=on  channel4=on  channel5=off  channel6=on  channel7=on  channel8=off  channel_count=off  rssi=off  rc_input_source=off  timestamp_last_signal=off  time_stamp=off  sampleTime=-1  BlockingMode=off  BlockTimeout=5
      settings: SourceProductBaseCode=PX4AUTOPILOTS
  Scope3 : Scope  NumInputPorts=4
  Terminator : Terminator
  Terminator2 : Terminator
  kill sw : MATLAB Function  TreatAsAtomicUnit=on
  Out1 : Outport
  Out2 : Outport  Port=2
  Out3 : Outport  Port=3
  Out4 : Outport  Port=4
  Out5 : Outport  Port=5
  Out6 : Outport  Port=6
  Out7 : Outport  Port=7
  y : Outport  Port=8
  ch6 : Outport  Port=9
  tag scope: acc_yaw_sp=global, w_yaw_sp=global, yaw_sp=global
  wires:
  Mux2/1 -> Out3/1  "a_des"
  Mux1/1 -> Out2/1  "v_des"
  Mux/1 -> Out1/1  "x_des"
  Cast To Double2/1 -> Out6/1, Scope3/3  "thrust_rc"
  Cast To Double3/1 -> Scope3/4, Out7/1  "yaw_rc"
  Radio Control Transmitter/2 -> Cast To Double/1  "roll"
  Cast To Double1/1 -> Out5/1, Scope3/2  "pitch_rc"
  Radio Control Transmitter/3 -> Cast To Double1/1  "pitch"
  Cast To Double/1 -> Out4/1, Scope3/1  "roll_rc"
  Radio Control Transmitter/4 -> Cast To Double2/1  "thrust"
  Radio Control Transmitter/5 -> Cast To Double3/1  "yaw"
  Radio Control Transmitter/1 -> Terminator2/1
  Radio Control Transmitter/7 -> kill sw/1(cmd)
  kill sw/1(kill_sw) -> y/1  "kill_switch"
  PX4 uORB Read1/1 -> Terminator/1
  PX4 uORB Read1/2 -> Bus Selector/1
  Bus Selector/1 -> Demux/1  "<setpoints>"
  Demux/1 -> Mux/1
  Demux/2 -> Mux/2
  Demux/3 -> Mux/3
  Demux/4 -> Mux1/1
  Demux/5 -> Mux1/2
  Demux/6 -> Mux1/3
  Demux/7 -> Mux2/1
  Demux/8 -> Mux2/2
  Demux/9 -> Mux2/3
  Demux/10 -> [yaw_sp]  "yaw_sp"
  Demux/11 -> [w_yaw_sp]  "w_yaw_sp"
  Demux/12 -> [acc_yaw_sp]  "acc_yaw_sp"
  Radio Control Transmitter/6 -> ch6/1  "ch6"

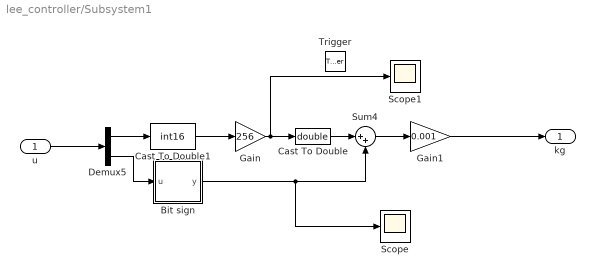
== system lee_controller/Subsystem1 ==
  u : Inport
  Trigger : TriggerPort  VariantControl=(inherit)  PortDimensions=1
  Bit sign : MATLAB Function  TreatAsAtomicUnit=on
  Cast To Double : DataTypeConversion  OutDataTypeStr=double
  Cast To Double1 : DataTypeConversion  OutDataTypeStr=int16
  Demux5 : Demux  Outputs=2
  Gain : Gain  Gain=256  OutDataTypeStr=int16
  Gain1 : Gain  Gain=0.001
  Scope : Scope
  Scope1 : Scope
  Sum4 : Sum  Inputs=|++
  kg : Outport
  wires:
  Gain1/1 -> kg/1
  Gain/1 -> Cast To Double/1, Scope1/1
  Sum4/1 -> Gain1/1
  Demux5/2 -> Bit sign/1(u)
  Bit sign/1(y) -> Scope/1, Sum4/2
  Demux5/1 -> Cast To Double1/1
  u/1 -> Demux5/1
  Cast To Double1/1 -> Gain/1
  Cast To Double/1 -> Sum4/1

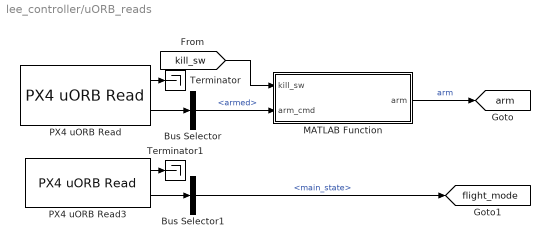
== system lee_controller/uORB_reads ==
  Bus Selector : BusSelector  OutputSignals=armed
  Bus Selector1 : BusSelector  OutputSignals=main_state
  MATLAB Function : MATLAB Function  TreatAsAtomicUnit=on
  PX4 uORB Read : px4uORBlib/PX4 uORB Read  uORBTopic=actuator_armed  selectInstance=actuator_armed  SampleTime=dt  BlockingMode=off  BlockTimeout=1e-3
      settings: SourceProductBaseCode=PX4AUTOPILOTS
  PX4 uORB Read3 : px4uORBlib/PX4 uORB Read  uORBTopic=commander_state  selectInstance=commander_state  SampleTime=dt  BlockingMode=off  BlockTimeout=1e-3
      settings: SourceProductBaseCode=PX4AUTOPILOTS
  Terminator : Terminator
  Terminator1 : Terminator
  tag scope: arm=global, flight_mode=global
  wires:
  Bus Selector1/1 -> [flight_mode]  "<main_state>"
  PX4 uORB Read3/1 -> Terminator1/1
  PX4 uORB Read/1 -> Terminator/1
  Bus Selector/1 -> MATLAB Function/2(arm_cmd)  "<armed>"
  MATLAB Function/1(arm) -> [arm]  "arm"
  [kill_sw] -> MATLAB Function/1(kill_sw)
  PX4 uORB Read/2 -> Bus Selector/1
  PX4 uORB Read3/2 -> Bus Selector1/1

== system lee_controller/Enabled Subsystem1/convert_thrust ==
  In1 : Inport
  Constant : Constant  Value=thrust_offset
  Data Type Conversion3 : DataTypeConversion  OutDataTypeStr=single
  Fcn6 : Fcn  Expr=(u - 1000) / 1000
  Saturation10 : Saturate  UpperLimit=1  LowerLimit=0
  Scope : Scope  NumInputPorts=2
  Sum : Sum  Inputs=|+-
  Out1 : Outport
  wires:
  Data Type Conversion3/1 -> Fcn6/1
  In1/1 -> Data Type Conversion3/1
  Saturation10/1 -> Out1/1
  Fcn6/1 -> Sum/1, Scope/1
  Sum/1 -> Scope/2, Saturation10/1
  Constant/1 -> Sum/2

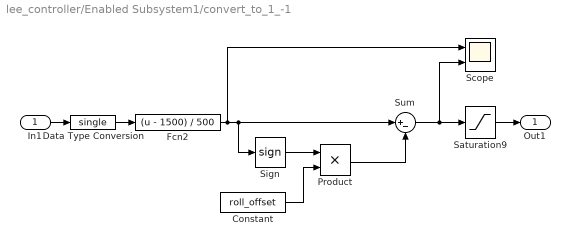
== system lee_controller/Enabled Subsystem1/convert_to_1_-1 ==
  In1 : Inport
  Constant : Constant  Value=roll_offset  SampleTime=-1
  Data Type Conversion : DataTypeConversion  OutDataTypeStr=single
  Fcn2 : Fcn  Expr=(u - 1500) / 500
  Product : Product
  Saturation9 : Saturate  UpperLimit=1  LowerLimit=-1
  Scope : Scope  NumInputPorts=2
  Sign : Signum
  Sum : Sum  Inputs=|+-
  Out1 : Outport
  wires:
  Fcn2/1 -> Sign/1, Sum/1, Scope/1
  Data Type Conversion/1 -> Fcn2/1
  Saturation9/1 -> Out1/1
  In1/1 -> Data Type Conversion/1
  Sum/1 -> Saturation9/1, Scope/2
  Constant/1 -> Product/2
  Sign/1 -> Product/1
  Product/1 -> Sum/2

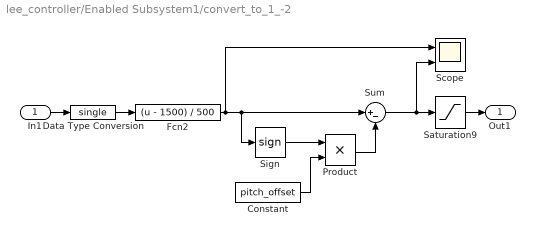
== system lee_controller/Enabled Subsystem1/convert_to_1_-2 ==
  In1 : Inport
  Constant : Constant  Value=pitch_offset  SampleTime=-1
  Data Type Conversion : DataTypeConversion  OutDataTypeStr=single
  Fcn2 : Fcn  Expr=(u - 1500) / 500
  Product : Product
  Saturation9 : Saturate  UpperLimit=1  LowerLimit=-1
  Scope : Scope  NumInputPorts=2
  Sign : Signum
  Sum : Sum  Inputs=|+-
  Out1 : Outport
  wires:
  In1/1 -> Data Type Conversion/1
  Saturation9/1 -> Out1/1
  Data Type Conversion/1 -> Fcn2/1
  Fcn2/1 -> Sign/1, Sum/1, Scope/1
  Sum/1 -> Scope/2, Saturation9/1
  Sign/1 -> Product/1
  Constant/1 -> Product/2
  Product/1 -> Sum/2

== system lee_controller/Enabled Subsystem1/convert_to_1_-3 ==
  In1 : Inport
  Constant : Constant  Value=yaw_offset  SampleTime=-1
  Data Type Conversion : DataTypeConversion  OutDataTypeStr=single
  Fcn2 : Fcn  Expr=(u - 1500) / 500
  Product : Product
  Saturation9 : Saturate  UpperLimit=1  LowerLimit=-1
  Scope : Scope  NumInputPorts=2
  Sign : Signum
  Sum : Sum  Inputs=|+-
  Out1 : Outport
  wires:
  Fcn2/1 -> Sign/1, Sum/1, Scope/1
  Data Type Conversion/1 -> Fcn2/1
  Saturation9/1 -> Out1/1
  In1/1 -> Data Type Conversion/1
  Sum/1 -> Scope/2, Saturation9/1
  Sign/1 -> Product/1
  Constant/1 -> Product/2
  Product/1 -> Sum/2

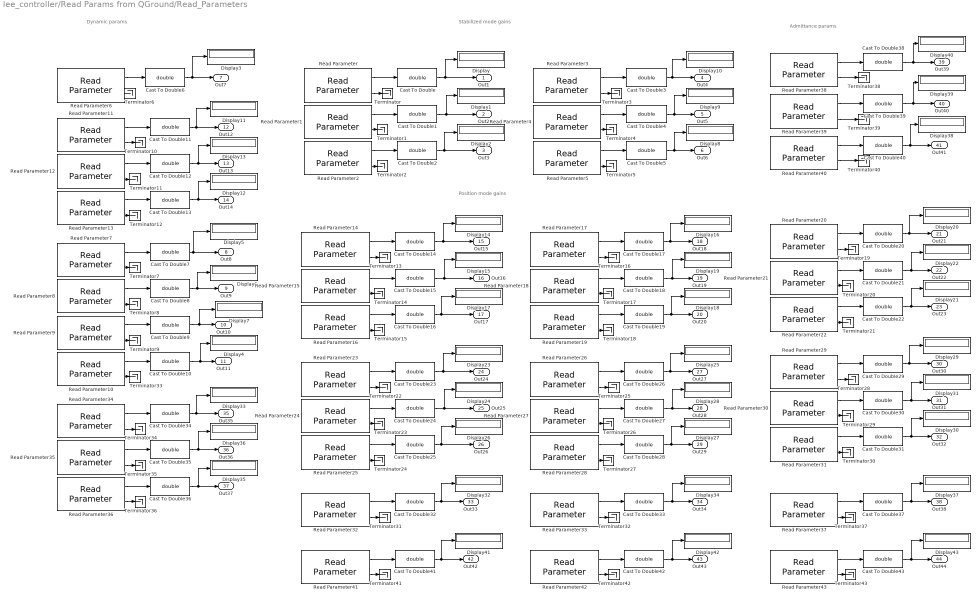
== system lee_controller/Read Params from QGround/Read_Parameters ==
  note: Stabilized mode gains
  note: Position mode gains
  note: Dynamic params
  note: Admittance params
  Cast To Double{,1..43} (44 alike) : DataTypeConversion  OutDataTypeStr=double
  Display{,1..43} (44 alike) : Display
  Read Parameter : px4lib/Read Parameter  ParameterName=LEE_KP_X_ATT  DataType=FLOAT  SampleTime=dt
      settings: SourceProductBaseCode=PX4AUTOPILOTS
  Read Parameter1 : px4lib/Read Parameter  ParameterName=LEE_KP_Y_ATT  DataType=FLOAT  SampleTime=dt
      settings: SourceProductBaseCode=PX4AUTOPILOTS
  Read Parameter10 : px4lib/Read Parameter  ParameterName=LEE_THRUST_MAX  DataType=FLOAT  SampleTime=dt
      settings: SourceProductBaseCode=PX4AUTOPILOTS
  Read Parameter11 : px4lib/Read Parameter  ParameterName=LEE_J_XX  DataType=FLOAT  SampleTime=dt
      settings: SourceProductBaseCode=PX4AUTOPILOTS
  Read Parameter12 : px4lib/Read Parameter  ParameterName=LEE_J_YY  DataType=FLOAT  SampleTime=dt
      settings: SourceProductBaseCode=PX4AUTOPILOTS
  Read Parameter13 : px4lib/Read Parameter  ParameterName=LEE_J_ZZ  DataType=FLOAT  SampleTime=dt
      settings: SourceProductBaseCode=PX4AUTOPILOTS
  Read Parameter14 : px4lib/Read Parameter  ParameterName=LEE_KP_X_POS  DataType=FLOAT  SampleTime=dt
      settings: SourceProductBaseCode=PX4AUTOPILOTS
  Read Parameter15 : px4lib/Read Parameter  ParameterName=LEE_KP_Y_POS  DataType=FLOAT  SampleTime=dt
      settings: SourceProductBaseCode=PX4AUTOPILOTS
  Read Parameter16 : px4lib/Read Parameter  ParameterName=LEE_KP_Z_POS  DataType=FLOAT  SampleTime=dt
      settings: SourceProductBaseCode=PX4AUTOPILOTS
  Read Parameter17 : px4lib/Read Parameter  ParameterName=LEE_KD_X_POS  DataType=FLOAT  SampleTime=dt
      settings: SourceProductBaseCode=PX4AUTOPILOTS
  Read Parameter18 : px4lib/Read Parameter  ParameterName=LEE_KD_Y_POS  DataType=FLOAT  SampleTime=dt
      settings: SourceProductBaseCode=PX4AUTOPILOTS
  Read Parameter19 : px4lib/Read Parameter  ParameterName=LEE_KD_Z_POS  DataType=FLOAT  SampleTime=dt
      settings: SourceProductBaseCode=PX4AUTOPILOTS
  Read Parameter2 : px4lib/Read Parameter  ParameterName=LEE_KP_Z_ATT  DataType=FLOAT  SampleTime=dt
      settings: SourceProductBaseCode=PX4AUTOPILOTS
  Read Parameter20 : px4lib/Read Parameter  ParameterName=LEE_KI_X_POS  DataType=FLOAT  SampleTime=dt
      settings: SourceProductBaseCode=PX4AUTOPILOTS
  Read Parameter21 : px4lib/Read Parameter  ParameterName=LEE_KI_Y_POS  DataType=FLOAT  SampleTime=dt
      settings: SourceProductBaseCode=PX4AUTOPILOTS
  Read Parameter22 : px4lib/Read Parameter  ParameterName=LEE_KI_Z_POS  DataType=FLOAT  SampleTime=dt
      settings: SourceProductBaseCode=PX4AUTOPILOTS
  Read Parameter23 : px4lib/Read Parameter  ParameterName=LEE_KP_X_OR  DataType=FLOAT  SampleTime=dt
      settings: SourceProductBaseCode=PX4AUTOPILOTS
  Read Parameter24 : px4lib/Read Parameter  ParameterName=LEE_KP_Y_OR  DataType=FLOAT  SampleTime=dt
      settings: SourceProductBaseCode=PX4AUTOPILOTS
  Read Parameter25 : px4lib/Read Parameter  ParameterName=LEE_KP_Z_OR  DataType=FLOAT  SampleTime=dt
      settings: SourceProductBaseCode=PX4AUTOPILOTS
  Read Parameter26 : px4lib/Read Parameter  ParameterName=LEE_KD_X_OR  DataType=FLOAT  SampleTime=dt
      settings: SourceProductBaseCode=PX4AUTOPILOTS
  Read Parameter27 : px4lib/Read Parameter  ParameterName=LEE_KD_Y_OR  DataType=FLOAT  SampleTime=dt
      settings: SourceProductBaseCode=PX4AUTOPILOTS
  Read Parameter28 : px4lib/Read Parameter  ParameterName=LEE_KD_Z_OR  DataType=FLOAT  SampleTime=dt
      settings: SourceProductBaseCode=PX4AUTOPILOTS
  Read Parameter29 : px4lib/Read Parameter  ParameterName=LEE_KI_X_OR  DataType=FLOAT  SampleTime=dt
      settings: SourceProductBaseCode=PX4AUTOPILOTS
  Read Parameter3 : px4lib/Read Parameter  ParameterName=LEE_KD_X_ATT  DataType=FLOAT  SampleTime=dt
      settings: SourceProductBaseCode=PX4AUTOPILOTS
  Read Parameter30 : px4lib/Read Parameter  ParameterName=LEE_KI_Y_OR  DataType=FLOAT  SampleTime=dt
      settings: SourceProductBaseCode=PX4AUTOPILOTS
  Read Parameter31 : px4lib/Read Parameter  ParameterName=LEE_KI_Z_OR  DataType=FLOAT  SampleTime=dt
      settings: SourceProductBaseCode=PX4AUTOPILOTS
  Read Parameter32 : px4lib/Read Parameter  ParameterName=LEE_C1  DataType=FLOAT  SampleTime=dt
      settings: SourceProductBaseCode=PX4AUTOPILOTS
  Read Parameter33 : px4lib/Read Parameter  ParameterName=LEE_C2  DataType=FLOAT  SampleTime=dt
      settings: SourceProductBaseCode=PX4AUTOPILOTS
  Read Parameter34 : px4lib/Read Parameter  ParameterName=LEE_KF  DataType=FLOAT  SampleTime=dt
      settings: SourceProductBaseCode=PX4AUTOPILOTS
  Read Parameter35 : px4lib/Read Parameter  ParameterName=LEE_KM  DataType=FLOAT  SampleTime=dt
      settings: SourceProductBaseCode=PX4AUTOPILOTS
  Read Parameter36 : px4lib/Read Parameter  ParameterName=LEE_L_ARM  DataType=FLOAT  SampleTime=dt
      settings: SourceProductBaseCode=PX4AUTOPILOTS
  Read Parameter37 : px4lib/Read Parameter  ParameterName=LEE_SAT_INT_ACT  DataType=FLOAT  SampleTime=dt
      settings: SourceProductBaseCode=PX4AUTOPILOTS
  Read Parameter38 : px4lib/Read Parameter  ParameterName=KP_A  DataType=FLOAT  SampleTime=dt
      settings: SourceProductBaseCode=PX4AUTOPILOTS
  Read Parameter39 : px4lib/Read Parameter  ParameterName=KD_A  DataType=FLOAT  SampleTime=dt
      settings: SourceProductBaseCode=PX4AUTOPILOTS
  Read Parameter4 : px4lib/Read Parameter  ParameterName=LEE_KD_Y_ATT  DataType=FLOAT  SampleTime=dt
      settings: SourceProductBaseCode=PX4AUTOPILOTS
  Read Parameter40 : px4lib/Read Parameter  ParameterName=M_A  DataType=FLOAT  SampleTime=dt
      settings: SourceProductBaseCode=PX4AUTOPILOTS
  Read Parameter41 : px4lib/Read Parameter  ParameterName=NED_Z  DataType=FLOAT  SampleTime=dt
      settings: SourceProductBaseCode=PX4AUTOPILOTS
  Read Parameter42 : px4lib/Read Parameter  ParameterName=NED_DZ  DataType=FLOAT  SampleTime=dt
      settings: SourceProductBaseCode=PX4AUTOPILOTS
  Read Parameter43 : px4lib/Read Parameter  ParameterName=NED_DDZ  DataType=FLOAT  SampleTime=dt
      settings: SourceProductBaseCode=PX4AUTOPILOTS
  Read Parameter5 : px4lib/Read Parameter  ParameterName=LEE_KD_Z_ATT  DataType=FLOAT  SampleTime=dt
      settings: SourceProductBaseCode=PX4AUTOPILOTS
  Read Parameter6 : px4lib/Read Parameter  ParameterName=LEE_MASS  DataType=FLOAT  SampleTime=dt
      settings: SourceProductBaseCode=PX4AUTOPILOTS
  Read Parameter7 : px4lib/Read Parameter  ParameterName=LEE_ROLL_MAX  DataType=FLOAT  SampleTime=dt
      settings: SourceProductBaseCode=PX4AUTOPILOTS
  Read Parameter8 : px4lib/Read Parameter  ParameterName=LEE_PITCH_MAX  DataType=FLOAT  SampleTime=dt
      settings: SourceProductBaseCode=PX4AUTOPILOTS
  Read Parameter9 : px4lib/Read Parameter  ParameterName=LEE_YAW_RATE_MAX  DataType=FLOAT  SampleTime=dt
      settings: SourceProductBaseCode=PX4AUTOPILOTS
  Terminator{,1..43} (44 alike) : Terminator
  Out1 : Outport
  Out2 : Outport  Port=2
  Out3 : Outport  Port=3
  Out4 : Outport  Port=4
  Out5 : Outport  Port=5
  Out6 : Outport  Port=6
  Out7 : Outport  Port=7
  Out8 : Outport  Port=8
  Out9 : Outport  Port=9
  Out10 : Outport  Port=10
  Out11 : Outport  Port=11
  Out12 : Outport  Port=12
  Out13 : Outport  Port=13
  Out14 : Outport  Port=14
  Out15 : Outport  Port=15
  Out16 : Outport  Port=16
  Out17 : Outport  Port=17
  Out18 : Outport  Port=18
  Out19 : Outport  Port=19
  Out20 : Outport  Port=20
  Out21 : Outport  Port=21
  Out22 : Outport  Port=22
  Out23 : Outport  Port=23
  Out24 : Outport  Port=24
  Out25 : Outport  Port=25
  Out26 : Outport  Port=26
  Out27 : Outport  Port=27
  Out28 : Outport  Port=28
  Out29 : Outport  Port=29
  Out30 : Outport  Port=30
  Out31 : Outport  Port=31
  Out32 : Outport  Port=32
  Out33 : Outport  Port=33
  Out34 : Outport  Port=34
  Out35 : Outport  Port=35
  Out36 : Outport  Port=36
  Out37 : Outport  Port=37
  Out38 : Outport  Port=38
  Out39 : Outport  Port=39
  Out40 : Outport  Port=40
  Out41 : Outport  Port=41
  Out42 : Outport  Port=42
  Out43 : Outport  Port=43
  Out44 : Outport  Port=44
  wires:
  Read Parameter/2 -> Terminator/1
  Read Parameter/1 -> Cast To Double/1
  Cast To Double/1 -> Out1/1, Display/1
  Cast To Double1/1 -> Out2/1, Display1/1
  Read Parameter1/1 -> Cast To Double1/1
  Cast To Double2/1 -> Out3/1, Display2/1
  Read Parameter2/1 -> Cast To Double2/1
  Read Parameter2/2 -> Terminator2/1
  Read Parameter1/2 -> Terminator1/1
  Read Parameter4/2 -> Terminator4/1
  Read Parameter5/2 -> Terminator5/1
  Read Parameter5/1 -> Cast To Double5/1
  Cast To Double5/1 -> Out6/1, Display8/1
  Read Parameter4/1 -> Cast To Double4/1
  Cast To Double4/1 -> Out5/1, Display9/1
  Cast To Double3/1 -> Out4/1, Display10/1
  Read Parameter3/1 -> Cast To Double3/1
  Read Parameter3/2 -> Terminator3/1
  Read Parameter6/2 -> Terminator6/1
  Read Parameter6/1 -> Cast To Double6/1
  Cast To Double6/1 -> Out7/1, Display3/1
  Read Parameter7/2 -> Terminator7/1
  Read Parameter7/1 -> Cast To Double7/1
  Cast To Double7/1 -> Out8/1, Display5/1
  Cast To Double8/1 -> Out9/1, Display6/1
  Read Parameter8/1 -> Cast To Double8/1
  Cast To Double9/1 -> Out10/1, Display7/1
  Read Parameter9/1 -> Cast To Double9/1
  Read Parameter9/2 -> Terminator9/1
  Read Parameter8/2 -> Terminator8/1
  Read Parameter10/1 -> Cast To Double10/1
  Cast To Double10/1 -> Out11/1, Display4/1
  Read Parameter11/2 -> Terminator10/1
  Read Parameter11/1 -> Cast To Double11/1
  Cast To Double11/1 -> Display11/1, Out12/1
  Cast To Double12/1 -> Display13/1, Out13/1
  Read Parameter12/1 -> Cast To Double12/1
  Cast To Double13/1 -> Display12/1, Out14/1
  Read Parameter13/1 -> Cast To Double13/1
  Read Parameter12/2 -> Terminator11/1
  Read Parameter13/2 -> Terminator12/1
  Read Parameter14/1 -> Cast To Double14/1
  Read Parameter18/1 -> Cast To Double18/1
  Read Parameter15/1 -> Cast To Double15/1
  Read Parameter19/1 -> Cast To Double19/1
  Cast To Double15/1 -> Out16/1, Display15/1
  Read Parameter16/1 -> Cast To Double16/1
  Read Parameter18/2 -> Terminator17/1
  Cast To Double16/1 -> Out17/1, Display17/1
  Read Parameter14/2 -> Terminator13/1
  Read Parameter16/2 -> Terminator15/1
  Cast To Double19/1 -> Out20/1, Display18/1
  Read Parameter17/1 -> Cast To Double17/1
  Read Parameter17/2 -> Terminator16/1
  Read Parameter15/2 -> Terminator14/1
  Cast To Double14/1 -> Out15/1, Display14/1
  Read Parameter19/2 -> Terminator18/1
  Cast To Double17/1 -> Out18/1, Display16/1
  Cast To Double18/1 -> Out19/1, Display19/1
  Read Parameter20/1 -> Cast To Double20/1
  Cast To Double22/1 -> Out23/1, Display21/1
  Read Parameter22/1 -> Cast To Double22/1
  Read Parameter21/2 -> Terminator20/1
  Read Parameter22/2 -> Terminator21/1
  Cast To Double21/1 -> Out22/1, Display22/1
  Read Parameter21/1 -> Cast To Double21/1
  Cast To Double20/1 -> Out21/1, Display20/1
  Read Parameter20/2 -> Terminator19/1
  Read Parameter24/2 -> Terminator23/1
  Read Parameter25/2 -> Terminator24/1
  Read Parameter31/1 -> Cast To Double31/1
  Cast To Double23/1 -> Out24/1, Display23/1
  Cast To Double24/1 -> Out25/1, Display24/1
  Cast To Double27/1 -> Out28/1, Display28/1
  Read Parameter28/2 -> Terminator27/1
  Read Parameter26/2 -> Terminator25/1
  Cast To Double26/1 -> Out27/1, Display25/1
  Read Parameter23/1 -> Cast To Double23/1
  Read Parameter24/1 -> Cast To Double24/1
  Read Parameter27/2 -> Terminator26/1
  Read Parameter29/2 -> Terminator28/1
  Read Parameter30/2 -> Terminator29/1
  Cast To Double29/1 -> Out30/1, Display29/1
  Cast To Double25/1 -> Out26/1, Display26/1
  Read Parameter23/2 -> Terminator22/1
  Cast To Double31/1 -> Out32/1, Display30/1
  Read Parameter25/1 -> Cast To Double25/1
  Read Parameter31/2 -> Terminator30/1
  Cast To Double30/1 -> Out31/1, Display31/1
  Cast To Double28/1 -> Out29/1, Display27/1
  Read Parameter27/1 -> Cast To Double27/1
  Read Parameter26/1 -> Cast To Double26/1
  Read Parameter28/1 -> Cast To Double28/1
  Read Parameter29/1 -> Cast To Double29/1
  Read Parameter30/1 -> Cast To Double30/1
  Read Parameter32/1 -> Cast To Double32/1
  Cast To Double32/1 -> Out33/1, Display32/1
  Read Parameter33/1 -> Cast To Double33/1
  Cast To Double33/1 -> Out34/1, Display34/1
  Read Parameter32/2 -> Terminator31/1
  Read Parameter33/2 -> Terminator32/1
  Read Parameter10/2 -> Terminator33/1
  Read Parameter36/2 -> Terminator36/1
  Read Parameter35/2 -> Terminator35/1
  Read Parameter36/1 -> Cast To Double36/1
  Cast To Double36/1 -> Out37/1, Display35/1
  Read Parameter35/1 -> Cast To Double35/1
  Cast To Double35/1 -> Out36/1, Display36/1
  Cast To Double34/1 -> Out35/1, Display33/1
  Read Parameter34/1 -> Cast To Double34/1
  Read Parameter34/2 -> Terminator34/1
  Cast To Double37/1 -> Display37/1, Out38/1
  Read Parameter37/1 -> Cast To Double37/1
  Read Parameter37/2 -> Terminator37/1
  Read Parameter40/2 -> Terminator40/1
  Read Parameter38/1 -> Cast To Double38/1
  Read Parameter39/1 -> Cast To Double39/1
  Read Parameter40/1 -> Cast To Double40/1
  Read Parameter39/2 -> Terminator39/1
  Read Parameter38/2 -> Terminator38/1
  Cast To Double39/1 -> Out40/1, Display39/1
  Cast To Double40/1 -> Out41/1, Display38/1
  Cast To Double38/1 -> Out39/1, Display40/1
  Read Parameter43/2 -> Terminator43/1
  Read Parameter43/1 -> Cast To Double43/1
  Cast To Double43/1 -> Out44/1, Display43/1
  Read Parameter42/2 -> Terminator42/1
  Read Parameter41/2 -> Terminator41/1
  Cast To Double42/1 -> Display42/1, Out43/1
  Read Parameter42/1 -> Cast To Double42/1
  Cast To Double41/1 -> Display41/1, Out42/1
  Read Parameter41/1 -> Cast To Double41/1

== matlab function lee_controller/LEE_CONTROLLER/inv alloc_matrix ==
  data: kf input; inv_A output; km input; l_arm input
function inv_A  = fcn(kf,km,l_arm)

    inv_A = [-1/(4*kf), -2^(1/2)/(4*l_arm*kf),  2^(1/2)/(4*l_arm*kf),  1/(4*km);
             -1/(4*kf),  2^(1/2)/(4*l_arm*kf), -2^(1/2)/(4*l_arm*kf),  1/(4*km);
             -1/(4*kf),  2^(1/2)/(4*l_arm*kf),  2^(1/2)/(4*l_arm*kf), -1/(4*km);
             -1/(4*kf), -2^(1/2)/(4*l_arm*kf), -2^(1/2)/(4*l_arm*kf), -1/(4*km)];
end

== matlab function lee_controller/LEE_CONTROLLER/MATLAB Function4 ==
  data: w_yaw_sp input; omega_d output; acc_yaw_sp input; omega_dd output
function [omega_d,omega_dd] = fcn(w_yaw_sp, acc_yaw_sp)

omega_d = [0,0,w_yaw_sp]';
omega_dd = [0,0,acc_yaw_sp]';
